simulink model "inverter_synth"  (R2020a)
settings: Solver=VariableStepAuto  StartTime=0.0  StopTime=0.75  MaxStep=0.001  RelTol=1e-4  EnableMultiTasking=on
model workspace (MAT data in the model file):
  f0 = 50
undefined symbols (not defined in the file): L, Lf, R, ron
libraries: powerlib x34, simulink_extras x9, powerlib_meascontrol x6, eeTransforms x5, simulink x5
settings Model: Creator=vm-user  LastModifiedBy=suku
settings DataIOCC: LimitDataPoints=on  SaveOutput=off  SaveTime=off  ReturnWorkspaceOutputs=off
settings OptimizationCC: ExpressionDepthLimit=2147483647  LifeSpan=1
settings DebuggingCC: UnderspecifiedInitializationDetection=Classic  MergeDetectMultiDrivingBlocksExec=none  FcnCallInpInsideContextMsg=warning  AllowSymbolicDim=off  StateNameClashWarn=warning  SFUnexpectedBacktrackingDiag=warning  SFNoUnconditionalDefaultTransitionDiag=warning  SFExecutionAtInitializationDiag=none  ArithmeticOperatorsInVariantConditions=warning
settings SFSimCC: SimUseLocalCustomCode=off  CustomCodeUndefinedFunction=UseInterfaceOnly
settings RTWCC: RTWUseLocalCustomCode=off
settings CodeAppCC: StateflowObjectComments=on
settings GRTTargetCC: TargetLangStandard=C89/C90 (ANSI)  CombineOutputUpdateFcns=off  GRTInterface=on

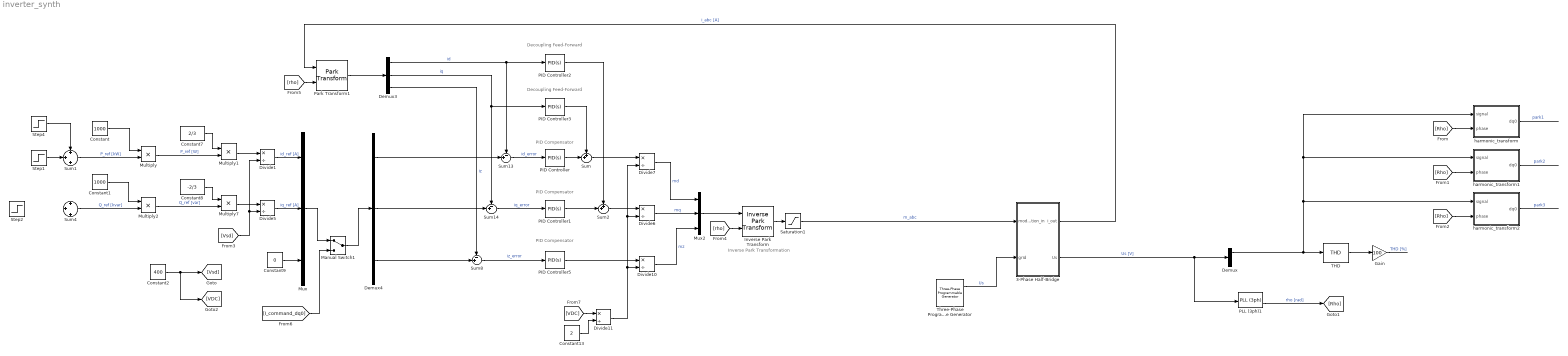
== system inverter_synth ==
  note: PID Compensator
  note: Decoupling Feed-Forward
  note: PID Compensator
  note: Decoupling Feed-Forward
  note: Inverse Park Transformation
  note: PID Compensator
  3-Phase Half-Bridge : Subsystem
  Constant : Constant  Value=1000
  Constant1 : Constant  Value=1000
  Constant13 : Constant  Value=2
  Constant2 : Constant  Value=400
  Constant7 : Constant  Value=2/3
  Constant8 : Constant  Value=-2/3
  Constant9 : Constant  Value=0
  Demux : Demux  Outputs=3
  Demux3 : Demux  Outputs=3
  Demux4 : Demux  Outputs=3
  Divide{1,5..7,10..11} (6 alike) : Product  Inputs=*/
  Gain : Gain  Gain=100
  Inverse Park Transform : eeTransforms/Inverse Park Transform  AxisAlignment=Q-axis  PowerInvariant=off
  Manual Switch1 : ManualSwitch
  Multiply{,1..2,7} (4 alike) : Product
  Mux : Mux  Inputs=3
  Mux2 : Mux  Inputs=3
  PID Controller : simulink/Continuous/PID Controller  Controller=PID  Form=Parallel  TimeDomain=Continuous-time  UseExternalTs=off  SampleTime=-1  IntegratorMethod=Forward Euler  FilterMethod=Forward Euler  ControllerParametersSource=internal  P=1  I=100  D=0.25  UseFilter=on  N=100  TunerSelectOption=Transfer Function Based (PID Tuner App)  InitialConditionSource=internal  InitialConditionForIntegrator=0  InitialConditionForFilter=0  DifferentiatorICPrevScaledInput=0  ExternalReset=none  TrackingMode=off  Kt=1  LimitOutput=off  UpperSaturationLimit=inf  LowerSaturationLimit=-inf  LinearizeAsGain=on  AntiWindupMode=none  Kb=1  POutMin=[]  POutMax=[]  IOutMin=[]  IOutMax=[]  DOutMin=[]  DOutMax=[]  NOutMin=[]  NOutMax=[]  SumOutMin=[]  SumOutMax=[]  SaturationOutMin=[]  SaturationOutMax=[]  PParamMin=[]  PParamMax=[]  IParamMin=[]  IParamMax=[]  DParamMin=[]  DParamMax=[]  NParamMin=[]  NParamMax=[]  KbParamMin=[]  KbParamMax=[]  KtParamMin=[]  KtParamMax=[]  KbOutMin=[]  KbOutMax=[]  KtOutMin=[]  KtOutMax=[]  IntegratorOutMin=[]  IntegratorOutMax=[]  FilterOutMin=[]  FilterOutMax=[]  SumI1OutMin=[]  SumI1OutMax=[]  SumI2OutMin=[]  SumI2OutMax=[]  SumI3OutMin=[]  SumI3OutMax=[]  SumI4OutMin=[]  SumI4OutMax=[]  SumDOutMin=[]  SumDOutMax=[]  DifferentiatorOutMin=[]  DifferentiatorOutMax=[]  FilterDiffOutCoefMin=[]  FilterDiffOutCoefMax=[]  ReciprocalOutMin=[]  ReciprocalOutMax=[]  SumDenOutMin=[]  SumDenOutMax=[]  SumNumOutMin=[]  SumNumOutMax=[]  DivideOutMin=[]  DivideOutMax=[]  UdiffTsProdOutMin=[]  UdiffTsProdOutMax=[]  NTsProdOutMin=[]  NTsProdOutMax=[]  UintegralTsProdOutMin=[]  UintegralTsProdOutMax=[]  UngainTsProdOutMin=[]  UngainTsProdOutMax=[]  IntegratorContinuousStateAttributes=''  IntegratorStateMustResolveToSignalObject=off  IntegratorRTWStateStorageClass=Auto  FilterContinuousStateAttributes=''  FilterStateMustResolveToSignalObject=off  FilterRTWStateStorageClass=Auto  ParallelPVariant=InternalParameters  IdealPVariant=Disabled  IVariant=InternalParameters  DVariant=InternalParameters  IntegratorVariant=Continuous  SatVariant=Disabled  AWVariant=Passthrough  PCopyVariant=Disabled  TRVariant=Disabled  FdbkBlocksVariant=Forward  IdealPFdbkVariant=Disabled  SatFdbkVariant=Disabled  DerivativeFilterVariant=ContFilter  NVariant=InternalParameters  NCopyVariant=Disabled  FilterICVariant=InternalICsFilter  IntegratorICVariant=InternalICs  ExternalResetVariant=Disabled  TRSumVariant=Passthrough  SumFdbkVariant=Disabled  SumVariant=Sum_PID  TsampFilterVariant=InternalTs  TsampNgainVariant=Passthrough  TsampIntegralVariant=Passthrough
  PID Controller1 : simulink/Continuous/PID Controller  Controller=PID  Form=Parallel  TimeDomain=Continuous-time  UseExternalTs=off  SampleTime=-1  IntegratorMethod=Forward Euler  FilterMethod=Forward Euler  ControllerParametersSource=internal  P=1  I=100  D=0.25  UseFilter=on  N=100  TunerSelectOption=Transfer Function Based (PID Tuner App)  InitialConditionSource=internal  InitialConditionForIntegrator=0  InitialConditionForFilter=0  DifferentiatorICPrevScaledInput=0  ExternalReset=none  TrackingMode=off  Kt=1  LimitOutput=off  UpperSaturationLimit=inf  LowerSaturationLimit=-inf  LinearizeAsGain=on  AntiWindupMode=none  Kb=1  POutMin=[]  POutMax=[]  IOutMin=[]  IOutMax=[]  DOutMin=[]  DOutMax=[]  NOutMin=[]  NOutMax=[]  SumOutMin=[]  SumOutMax=[]  SaturationOutMin=[]  SaturationOutMax=[]  PParamMin=[]  PParamMax=[]  IParamMin=[]  IParamMax=[]  DParamMin=[]  DParamMax=[]  NParamMin=[]  NParamMax=[]  KbParamMin=[]  KbParamMax=[]  KtParamMin=[]  KtParamMax=[]  KbOutMin=[]  KbOutMax=[]  KtOutMin=[]  KtOutMax=[]  IntegratorOutMin=[]  IntegratorOutMax=[]  FilterOutMin=[]  FilterOutMax=[]  SumI1OutMin=[]  SumI1OutMax=[]  SumI2OutMin=[]  SumI2OutMax=[]  SumI3OutMin=[]  SumI3OutMax=[]  SumI4OutMin=[]  SumI4OutMax=[]  SumDOutMin=[]  SumDOutMax=[]  DifferentiatorOutMin=[]  DifferentiatorOutMax=[]  FilterDiffOutCoefMin=[]  FilterDiffOutCoefMax=[]  ReciprocalOutMin=[]  ReciprocalOutMax=[]  SumDenOutMin=[]  SumDenOutMax=[]  SumNumOutMin=[]  SumNumOutMax=[]  DivideOutMin=[]  DivideOutMax=[]  UdiffTsProdOutMin=[]  UdiffTsProdOutMax=[]  NTsProdOutMin=[]  NTsProdOutMax=[]  UintegralTsProdOutMin=[]  UintegralTsProdOutMax=[]  UngainTsProdOutMin=[]  UngainTsProdOutMax=[]  IntegratorContinuousStateAttributes=''  IntegratorStateMustResolveToSignalObject=off  IntegratorRTWStateStorageClass=Auto  FilterContinuousStateAttributes=''  FilterStateMustResolveToSignalObject=off  FilterRTWStateStorageClass=Auto  ParallelPVariant=InternalParameters  IdealPVariant=Disabled  IVariant=InternalParameters  DVariant=InternalParameters  IntegratorVariant=Continuous  SatVariant=Disabled  AWVariant=Passthrough  PCopyVariant=Disabled  TRVariant=Disabled  FdbkBlocksVariant=Forward  IdealPFdbkVariant=Disabled  SatFdbkVariant=Disabled  DerivativeFilterVariant=ContFilter  NVariant=InternalParameters  NCopyVariant=Disabled  FilterICVariant=InternalICsFilter  IntegratorICVariant=InternalICs  ExternalResetVariant=Disabled  TRSumVariant=Passthrough  SumFdbkVariant=Disabled  SumVariant=Sum_PID  TsampFilterVariant=InternalTs  TsampNgainVariant=Passthrough  TsampIntegralVariant=Passthrough
  PID Controller2 : simulink/Continuous/PID Controller  Controller=PID  Form=Parallel  TimeDomain=Continuous-time  UseExternalTs=off  SampleTime=-1  IntegratorMethod=Forward Euler  FilterMethod=Forward Euler  ControllerParametersSource=internal  P=0.22  I=0  D=0  UseFilter=on  N=100  TunerSelectOption=Transfer Function Based (PID Tuner App)  InitialConditionSource=internal  InitialConditionForIntegrator=0  InitialConditionForFilter=0  DifferentiatorICPrevScaledInput=0  ExternalReset=none  TrackingMode=off  Kt=1  LimitOutput=off  UpperSaturationLimit=inf  LowerSaturationLimit=-inf  LinearizeAsGain=on  AntiWindupMode=none  Kb=1  POutMin=[]  POutMax=[]  IOutMin=[]  IOutMax=[]  DOutMin=[]  DOutMax=[]  NOutMin=[]  NOutMax=[]  SumOutMin=[]  SumOutMax=[]  SaturationOutMin=[]  SaturationOutMax=[]  PParamMin=[]  PParamMax=[]  IParamMin=[]  IParamMax=[]  DParamMin=[]  DParamMax=[]  NParamMin=[]  NParamMax=[]  KbParamMin=[]  KbParamMax=[]  KtParamMin=[]  KtParamMax=[]  KbOutMin=[]  KbOutMax=[]  KtOutMin=[]  KtOutMax=[]  IntegratorOutMin=[]  IntegratorOutMax=[]  FilterOutMin=[]  FilterOutMax=[]  SumI1OutMin=[]  SumI1OutMax=[]  SumI2OutMin=[]  SumI2OutMax=[]  SumI3OutMin=[]  SumI3OutMax=[]  SumI4OutMin=[]  SumI4OutMax=[]  SumDOutMin=[]  SumDOutMax=[]  DifferentiatorOutMin=[]  DifferentiatorOutMax=[]  FilterDiffOutCoefMin=[]  FilterDiffOutCoefMax=[]  ReciprocalOutMin=[]  ReciprocalOutMax=[]  SumDenOutMin=[]  SumDenOutMax=[]  SumNumOutMin=[]  SumNumOutMax=[]  DivideOutMin=[]  DivideOutMax=[]  UdiffTsProdOutMin=[]  UdiffTsProdOutMax=[]  NTsProdOutMin=[]  NTsProdOutMax=[]  UintegralTsProdOutMin=[]  UintegralTsProdOutMax=[]  UngainTsProdOutMin=[]  UngainTsProdOutMax=[]  IntegratorContinuousStateAttributes=''  IntegratorStateMustResolveToSignalObject=off  IntegratorRTWStateStorageClass=Auto  FilterContinuousStateAttributes=''  FilterStateMustResolveToSignalObject=off  FilterRTWStateStorageClass=Auto  ParallelPVariant=InternalParameters  IdealPVariant=Disabled  IVariant=InternalParameters  DVariant=InternalParameters  IntegratorVariant=Continuous  SatVariant=Disabled  AWVariant=Passthrough  PCopyVariant=Disabled  TRVariant=Disabled  FdbkBlocksVariant=Forward  IdealPFdbkVariant=Disabled  SatFdbkVariant=Disabled  DerivativeFilterVariant=ContFilter  NVariant=InternalParameters  NCopyVariant=Disabled  FilterICVariant=InternalICsFilter  IntegratorICVariant=InternalICs  ExternalResetVariant=Disabled  TRSumVariant=Passthrough  SumFdbkVariant=Disabled  SumVariant=Sum_PID  TsampFilterVariant=InternalTs  TsampNgainVariant=Passthrough  TsampIntegralVariant=Passthrough
  PID Controller3 : simulink/Continuous/PID Controller  Controller=PID  Form=Parallel  TimeDomain=Continuous-time  UseExternalTs=off  SampleTime=-1  IntegratorMethod=Forward Euler  FilterMethod=Forward Euler  ControllerParametersSource=internal  P=-0.22  I=0  D=0  UseFilter=on  N=100  TunerSelectOption=Transfer Function Based (PID Tuner App)  InitialConditionSource=internal  InitialConditionForIntegrator=0  InitialConditionForFilter=0  DifferentiatorICPrevScaledInput=0  ExternalReset=none  TrackingMode=off  Kt=1  LimitOutput=off  UpperSaturationLimit=inf  LowerSaturationLimit=-inf  LinearizeAsGain=on  AntiWindupMode=none  Kb=1  POutMin=[]  POutMax=[]  IOutMin=[]  IOutMax=[]  DOutMin=[]  DOutMax=[]  NOutMin=[]  NOutMax=[]  SumOutMin=[]  SumOutMax=[]  SaturationOutMin=[]  SaturationOutMax=[]  PParamMin=[]  PParamMax=[]  IParamMin=[]  IParamMax=[]  DParamMin=[]  DParamMax=[]  NParamMin=[]  NParamMax=[]  KbParamMin=[]  KbParamMax=[]  KtParamMin=[]  KtParamMax=[]  KbOutMin=[]  KbOutMax=[]  KtOutMin=[]  KtOutMax=[]  IntegratorOutMin=[]  IntegratorOutMax=[]  FilterOutMin=[]  FilterOutMax=[]  SumI1OutMin=[]  SumI1OutMax=[]  SumI2OutMin=[]  SumI2OutMax=[]  SumI3OutMin=[]  SumI3OutMax=[]  SumI4OutMin=[]  SumI4OutMax=[]  SumDOutMin=[]  SumDOutMax=[]  DifferentiatorOutMin=[]  DifferentiatorOutMax=[]  FilterDiffOutCoefMin=[]  FilterDiffOutCoefMax=[]  ReciprocalOutMin=[]  ReciprocalOutMax=[]  SumDenOutMin=[]  SumDenOutMax=[]  SumNumOutMin=[]  SumNumOutMax=[]  DivideOutMin=[]  DivideOutMax=[]  UdiffTsProdOutMin=[]  UdiffTsProdOutMax=[]  NTsProdOutMin=[]  NTsProdOutMax=[]  UintegralTsProdOutMin=[]  UintegralTsProdOutMax=[]  UngainTsProdOutMin=[]  UngainTsProdOutMax=[]  IntegratorContinuousStateAttributes=''  IntegratorStateMustResolveToSignalObject=off  IntegratorRTWStateStorageClass=Auto  FilterContinuousStateAttributes=''  FilterStateMustResolveToSignalObject=off  FilterRTWStateStorageClass=Auto  ParallelPVariant=InternalParameters  IdealPVariant=Disabled  IVariant=InternalParameters  DVariant=InternalParameters  IntegratorVariant=Continuous  SatVariant=Disabled  AWVariant=Passthrough  PCopyVariant=Disabled  TRVariant=Disabled  FdbkBlocksVariant=Forward  IdealPFdbkVariant=Disabled  SatFdbkVariant=Disabled  DerivativeFilterVariant=ContFilter  NVariant=InternalParameters  NCopyVariant=Disabled  FilterICVariant=InternalICsFilter  IntegratorICVariant=InternalICs  ExternalResetVariant=Disabled  TRSumVariant=Passthrough  SumFdbkVariant=Disabled  SumVariant=Sum_PID  TsampFilterVariant=InternalTs  TsampNgainVariant=Passthrough  TsampIntegralVariant=Passthrough
  PID Controller5 : simulink/Continuous/PID Controller  Controller=PID  Form=Parallel  TimeDomain=Continuous-time  UseExternalTs=off  SampleTime=-1  IntegratorMethod=Forward Euler  FilterMethod=Forward Euler  ControllerParametersSource=internal  P=1  I=100  D=0.25  UseFilter=on  N=100  TunerSelectOption=Transfer Function Based (PID Tuner App)  InitialConditionSource=internal  InitialConditionForIntegrator=0  InitialConditionForFilter=0  DifferentiatorICPrevScaledInput=0  ExternalReset=none  TrackingMode=off  Kt=1  LimitOutput=off  UpperSaturationLimit=inf  LowerSaturationLimit=-inf  LinearizeAsGain=on  AntiWindupMode=none  Kb=1  POutMin=[]  POutMax=[]  IOutMin=[]  IOutMax=[]  DOutMin=[]  DOutMax=[]  NOutMin=[]  NOutMax=[]  SumOutMin=[]  SumOutMax=[]  SaturationOutMin=[]  SaturationOutMax=[]  PParamMin=[]  PParamMax=[]  IParamMin=[]  IParamMax=[]  DParamMin=[]  DParamMax=[]  NParamMin=[]  NParamMax=[]  KbParamMin=[]  KbParamMax=[]  KtParamMin=[]  KtParamMax=[]  KbOutMin=[]  KbOutMax=[]  KtOutMin=[]  KtOutMax=[]  IntegratorOutMin=[]  IntegratorOutMax=[]  FilterOutMin=[]  FilterOutMax=[]  SumI1OutMin=[]  SumI1OutMax=[]  SumI2OutMin=[]  SumI2OutMax=[]  SumI3OutMin=[]  SumI3OutMax=[]  SumI4OutMin=[]  SumI4OutMax=[]  SumDOutMin=[]  SumDOutMax=[]  DifferentiatorOutMin=[]  DifferentiatorOutMax=[]  FilterDiffOutCoefMin=[]  FilterDiffOutCoefMax=[]  ReciprocalOutMin=[]  ReciprocalOutMax=[]  SumDenOutMin=[]  SumDenOutMax=[]  SumNumOutMin=[]  SumNumOutMax=[]  DivideOutMin=[]  DivideOutMax=[]  UdiffTsProdOutMin=[]  UdiffTsProdOutMax=[]  NTsProdOutMin=[]  NTsProdOutMax=[]  UintegralTsProdOutMin=[]  UintegralTsProdOutMax=[]  UngainTsProdOutMin=[]  UngainTsProdOutMax=[]  IntegratorContinuousStateAttributes=''  IntegratorStateMustResolveToSignalObject=off  IntegratorRTWStateStorageClass=Auto  FilterContinuousStateAttributes=''  FilterStateMustResolveToSignalObject=off  FilterRTWStateStorageClass=Auto  ParallelPVariant=InternalParameters  IdealPVariant=Disabled  IVariant=InternalParameters  DVariant=InternalParameters  IntegratorVariant=Continuous  SatVariant=Disabled  AWVariant=Passthrough  PCopyVariant=Disabled  TRVariant=Disabled  FdbkBlocksVariant=Forward  IdealPFdbkVariant=Disabled  SatFdbkVariant=Disabled  DerivativeFilterVariant=ContFilter  NVariant=InternalParameters  NCopyVariant=Disabled  FilterICVariant=InternalICsFilter  IntegratorICVariant=InternalICs  ExternalResetVariant=Disabled  TRSumVariant=Passthrough  SumFdbkVariant=Disabled  SumVariant=Sum_PID  TsampFilterVariant=InternalTs  TsampNgainVariant=Passthrough  TsampIntegralVariant=Passthrough
  PLL (3ph)1 : powerlib_meascontrol/PLL/PLL (3ph)  Fmin=40  Par_Init=[0, 50]  ParK=[180, 3200, 1]  TcD=1e-4  MaxRateChangeFreq=12  FilterCutOffFreq=25  Ts=0  AGC=on
  Park Transform1 : eeTransforms/Park Transform  AxisAlignment=Q-axis  PowerInvariant=off
  Saturation1 : Saturate  UpperLimit=1  LowerLimit=-1
  Step1 : Step  Time=0.1  After=8  SampleTime=0
  Step2 : Step  Time=0.5  After=6  SampleTime=0
  Step4 : Step  Time=0.5  After=-4  SampleTime=0
  Sum : Sum  Inputs=++|
  Sum1 : Sum  Inputs=+|+|+
  Sum13 : Sum  Inputs=-+|
  Sum14 : Sum  Inputs=-+|
  Sum2 : Sum  Inputs=++|
  Sum4 : Sum  Inputs=+|+|+
  Sum8 : Sum  Inputs=-+|
  THD : powerlib_meascontrol/Measurements/THD  Freq=50  Ts=0
  Three-Phase Programmable Generator : powerlib_meascontrol/Pulse & Signal Generators/Three-Phase Programmable Generator  Par_Vps=[231, 0, 50]  VariationEntity=None  VariationType=Ramp  VariationStep=-0.5  VariationRate=10  VariationMag=0.3  VariationFreq=2  Par_Timing_Variation="[0.2  1.2]"  SinglePhase=on  Yampli=[1 0.2 1.2 1.0]  Xtime=[0 0.1 0.15 0.2]  HarmonicGeneration=on  Par_HarmoA="[3  50  25 0]"  Par_HarmoB="[5  30  -42  2]"  Par_Timing_Harmo="[ 0.05  99]"  Ts=0
      settings: SourceProductBaseCode=PS
  harmonic_transform : Subsystem  mask{f0=50, h=1}
      mask prompts: f0 "fundamental frequency"; h "harmonic number"
  harmonic_transform1 : Subsystem  mask{f0=50, h=3}
      mask prompts: f0 "fundamental frequency"; h "harmonic number"
  harmonic_transform2 : Subsystem  mask{f0=50, h=5}
      mask prompts: f0 "fundamental frequency"; h "harmonic number"
  wires:
  PLL (3ph)1/2 -> [Rho]  "rho [rad]"
  harmonic_transform/1(dq0) -> ?  "park1"
  [Rho] -> harmonic_transform/2(phase)
  [Rho] -> harmonic_transform1/2(phase)
  harmonic_transform1/1(dq0) -> ?  "park2"
  harmonic_transform2/1(dq0) -> ?  "park3"
  [Rho] -> harmonic_transform2/2(phase)
  Demux/1 -> harmonic_transform1/1(signal), harmonic_transform/1(signal), harmonic_transform2/1(signal), THD/1
  THD/1 -> Gain/1
  Gain/1 -> ?  "THD [%]"
  3-Phase Half-Bridge/2(Us) -> PLL (3ph)1/1, Demux/1  "Us [V]"
  Sum4/1 -> Multiply2/2  "Q_ref [kvar]"
  Demux4/1 -> Sum13/2
  Divide7/1 -> Mux2/1  "md"
  PID Controller2/1 -> Sum2/1
  Demux4/2 -> Sum14/2
  Demux3/3 -> Sum8/1  "iz"
  Sum8/1 -> PID Controller5/1  "iz_error"
  Constant7/1 -> Multiply1/1
  Constant9/1 -> Mux/3
  Sum14/1 -> PID Controller1/1  "iq_error"
  Divide1/1 -> Mux/1  "id_ref [A]"
  Sum2/1 -> Divide6/1
  Divide10/1 -> Mux2/3  "mz"
  Multiply7/1 -> Divide5/1
  [rho] -> Park Transform1/2
  Sum/1 -> Divide7/1
  PID Controller5/1 -> Divide10/1
  Manual Switch1/1 -> Demux4/1
  Divide6/1 -> Mux2/2  "mq"
  [rho] -> Inverse Park Transform/2
  Step1/1 -> Sum1/2
  PID Controller1/1 -> Sum2/2
  PID Controller3/1 -> Sum/1
  Step4/1 -> Sum1/1
  [VDC] -> Divide11/1
  3-Phase Half-Bridge/1(i_out) -> Park Transform1/1  "i_abc [A]"
  Demux3/2 -> Sum14/1, PID Controller3/1  "iq"
  Inverse Park Transform/1 -> Saturation1/1
  Divide11/1 -> Divide10/2, Divide7/2, Divide6/2
  Constant13/1 -> Divide11/2
  Constant1/1 -> Multiply2/1
  Multiply2/1 -> Multiply7/2  "Q_ref [var]"
  [Vsd] -> Divide1/2, Divide5/2
  Saturation1/1 -> 3-Phase Half-Bridge/1(modulation_in)  "m_abc"
  Multiply/1 -> Multiply1/2  "P_ref [W]"
  Demux3/1 -> Sum13/1, PID Controller2/1  "id"
  Mux/1 -> Manual Switch1/1
  Multiply1/1 -> Divide1/1
  Demux4/3 -> Sum8/2
  Constant/1 -> Multiply/1
  Sum13/1 -> PID Controller/1  "id_error"
  Divide5/1 -> Mux/2  "iq_ref [A]"
  Mux2/1 -> Inverse Park Transform/1
  [I_command_dq0] -> Manual Switch1/2
  Sum1/1 -> Multiply/2  "P_ref [kW]"
  Constant8/1 -> Multiply7/1
  PID Controller/1 -> Sum/2
  Park Transform1/1 -> Demux3/1
  Three-Phase Programmable Generator/1 -> 3-Phase Half-Bridge/2(grid)  "Us"
  Constant2/1 -> [VDC], [Vsd]

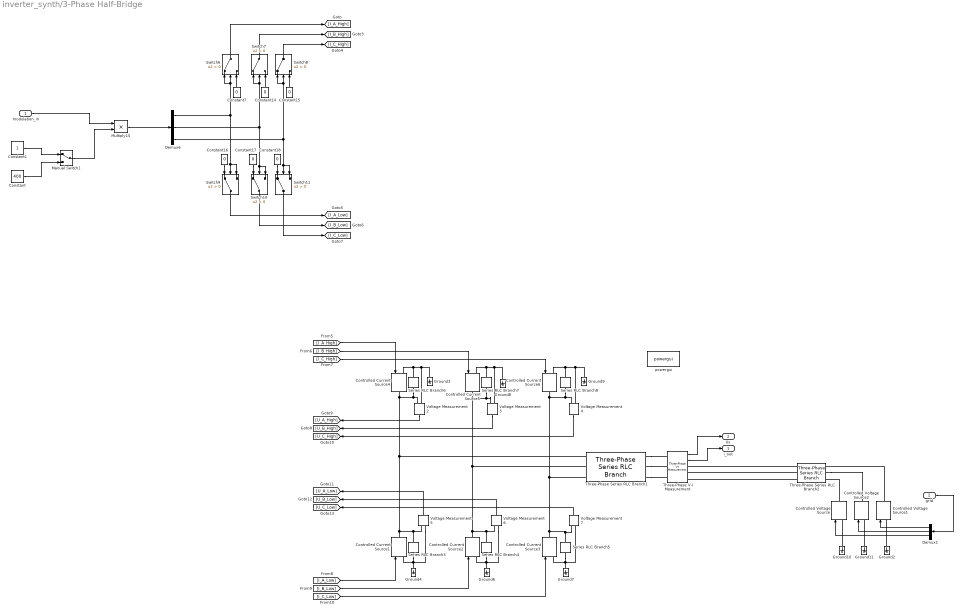
== system inverter_synth/3-Phase Half-Bridge ==
  modulation_in : Inport
  grid : Inport  Port=2
  Constant : Constant  Value=400
  Constant1 : Constant
  Constant{7,14..18} (6 alike) : Constant  Value=0
  Controlled Current Source{1..6} (6 alike) : powerlib/Electrical Sources/Controlled Current Source  Initialize=on  Source_Type=DC  Amplitude=0  Phase=0  Frequency=0  Measurements=None
  Controlled Voltage Source : powerlib/Electrical Sources/Controlled Voltage Source  Initialize=on  Source_Type=DC  Amplitude=0  Phase=0  Frequency=0  Measurements=None
  Controlled Voltage Source1 : powerlib/Electrical Sources/Controlled Voltage Source  Initialize=on  Source_Type=DC  Amplitude=0  Phase=0  Frequency=0  Measurements=None
  Controlled Voltage Source2 : powerlib/Electrical Sources/Controlled Voltage Source  Initialize=on  Source_Type=DC  Amplitude=0  Phase=0  Frequency=0  Measurements=None
  Demux1 : Demux  Outputs=3
  Demux6 : Demux  Outputs=3
  Ground{2..4,6..11} (9 alike) : powerlib/Elements/Ground  LConnTagsString=a
  Manual Switch1 : ManualSwitch
  Multiply15 : Product
  Series RLC Branch{3..8} (6 alike) : powerlib/Elements/Series RLC Branch  LConnTagsString=__new0  RConnTagsString=__new0  BranchType=R  Resistance=5000  Inductance=1e-3  SetiL0=off  InitialCurrent=0  Capacitance=47000e-6  Setx0=on  InitialVoltage=300  Measurements=None
  Switch{6..11} (6 alike) : Switch  Criteria=u2 > Threshold
  Three-Phase Series RLC Branch1 : powerlib/Elements/Three-Phase Series RLC Branch  LConnTagsString=A|B|C  RConnTagsString=A|B|C  BranchType=RL  Resistance=R + ron  Inductance=L  Capacitance=1e-6  Measurements=None
  Three-Phase Series RLC Branch2 : powerlib/Elements/Three-Phase Series RLC Branch  LConnTagsString=A|B|C  RConnTagsString=A|B|C  BranchType=RL  Resistance=1  Inductance=Lf  Capacitance=1e-6  Measurements=None
  Three-Phase V-I Measurement : powerlib/Measurements/Three-Phase V-I Measurement  VoltageMeasurement=phase-to-ground  SetLabelV=off  LabelV=Vabc  Vpu=off  VpuLL=off  CurrentMeasurement=yes  SetLabelI=off  LabelI=Iabc  Ipu=off  Pbase=100e6  Vbase=500e3  OutputType=Complex  PhasorSimulation=off  PSBequivalent=0
  Voltage Measurement{2..7} (6 alike) : powerlib/Measurements/Voltage Measurement  PhasorSimulation=off  OutputType=Magnitude  PSBequivalent=0
  powergui : powerlib/powergui  Priority=1  SimulationMode=Continuous  SampleTime=50e-6  frequency=60  Iterations=50  frequencyindice=0  Pbase=100e6  ErrMax=1e-4  UnitsV=kV  UnitsW=MW  buscounter=0  FunctionMessages=off  echomessages=off  EnableUseOfTLC=off  CurrentSourceSwitches=off  DisableSnubberDevices=off  DisableRonSwitches=off  DisableVfSwitches=off  DisplayEquations=off  AutomaticDiscreteSolvers=off  SolverType=Tustin/Backward Euler (TBE)  Interpol=off  ExternalGateDelay=off  methode=off  Ts=100  x0status=blocks  SPID=on  SwTol=0  HookPort=off  NonlinearTolerance=1e-4  nMaxIteration=100  ContinueOnMaxIteration=off  RestoreLinks=warning  ResistiveCurrentMeasurement=off  Frange=[0:2:500]  Ylog=off  Xlog=on  ShowGrid=off  save=off  variable=ZData  structure=0  ZoomFFT=off  StartTime=0.0  cycles=1  DisplayStyle=1  fundamental=60  FreqAxis=off  MaxFrequency=1000  frequencyindicesteady=1  RmsSteady=1  display=off
  i_out : Outport  VectorParamsAs1DForOutWhenUnconnected=off
  Us : Outport  Port=2  VectorParamsAs1DForOutWhenUnconnected=off
  wires:
  Constant18/1 -> Switch11/1
  Constant7/1 -> Switch6/3
  Constant16/1 -> Switch9/1
  Constant14/1 -> Switch7/3
  Constant17/1 -> Switch10/1
  Three-Phase V-I Measurement/2 -> i_out/1
  Constant15/1 -> Switch8/3
  Three-Phase V-I Measurement/1 -> Us/1
  modulation_in/1 -> Multiply15/1
  [I_A_High] -> Controlled Current Source4/1
  [I_B_High] -> Controlled Current Source5/1
  [I_C_High] -> Controlled Current Source6/1
  [I_B_Low] -> Controlled Current Source2/1
  [I_C_Low] -> Controlled Current Source3/1
  [I_A_Low] -> Controlled Current Source1/1
  Voltage Measurement2/1 -> [U_A_High]
  Voltage Measurement3/1 -> [U_B_High]
  Voltage Measurement4/1 -> [U_C_High]
  Voltage Measurement5/1 -> [U_A_Low]
  Voltage Measurement6/1 -> [U_B_Low]
  Voltage Measurement7/1 -> [U_C_Low]
  Switch8/1 -> [I_C_High]
  Switch7/1 -> [I_B_High]
  Switch6/1 -> [I_A_High]
  Switch11/1 -> [I_C_Low]
  Switch10/1 -> [I_B_Low]
  Switch9/1 -> [I_A_Low]
  Demux6/1 -> Switch6/1, Switch6/2, Switch9/3, Switch9/2
  Demux6/2 -> Switch7/1, Switch7/2, Switch10/3, Switch10/2
  Demux6/3 -> Switch11/3, Switch11/2, Switch8/1, Switch8/2
  Manual Switch1/1 -> Multiply15/2
  Constant/1 -> Manual Switch1/2
  Demux1/3 -> Controlled Voltage Source/1
  Demux1/2 -> Controlled Voltage Source2/1
  Demux1/1 -> Controlled Voltage Source1/1
  grid/1 -> Demux1/1
  Multiply15/1 -> Demux6/1
  Constant1/1 -> Manual Switch1/1
  connections:
  Controlled Current Source1/RConn1 -- Voltage Measurement5/LConn2 -- Series RLC Branch3/LConn1 -- Three-Phase Series RLC Branch1/LConn1 -- Voltage Measurement2/LConn2 -- Series RLC Branch6/RConn1 -- Controlled Current Source4/RConn1
  Controlled Current Source2/RConn1 -- Voltage Measurement6/LConn2 -- Series RLC Branch4/LConn1 -- Three-Phase Series RLC Branch1/LConn2 -- Voltage Measurement3/LConn2 -- Series RLC Branch7/RConn1 -- Controlled Current Source5/RConn1
  Controlled Current Source3/RConn1 -- Voltage Measurement7/LConn2 -- Series RLC Branch5/LConn1 -- Voltage Measurement4/LConn2 -- Series RLC Branch8/RConn1 -- Controlled Current Source6/RConn1 -- Three-Phase Series RLC Branch1/LConn3
  Three-Phase Series RLC Branch2/LConn1 -- Three-Phase V-I Measurement/RConn1
  Three-Phase Series RLC Branch2/LConn2 -- Three-Phase V-I Measurement/RConn2
  Three-Phase Series RLC Branch2/LConn3 -- Three-Phase V-I Measurement/RConn3
  Series RLC Branch4/RConn1 -- Voltage Measurement6/LConn1 -- Ground6/LConn1 -- Controlled Current Source2/LConn1
  Series RLC Branch3/RConn1 -- Voltage Measurement5/LConn1 -- Ground4/LConn1 -- Controlled Current Source1/LConn1
  Controlled Current Source5/LConn1 -- Ground8/LConn1 -- Voltage Measurement3/LConn1 -- Series RLC Branch7/LConn1
  Series RLC Branch5/RConn1 -- Ground7/LConn1 -- Controlled Current Source3/LConn1 -- Voltage Measurement7/LConn1
  Ground3/LConn1 -- Controlled Current Source4/LConn1 -- Series RLC Branch6/LConn1 -- Voltage Measurement2/LConn1
  Voltage Measurement4/LConn1 -- Controlled Current Source6/LConn1 -- Series RLC Branch8/LConn1 -- Ground9/LConn1
  Three-Phase Series RLC Branch1/RConn1 -- Three-Phase V-I Measurement/LConn1
  Three-Phase Series RLC Branch1/RConn2 -- Three-Phase V-I Measurement/LConn2
  Three-Phase Series RLC Branch1/RConn3 -- Three-Phase V-I Measurement/LConn3
  Three-Phase Series RLC Branch2/RConn2 -- Controlled Voltage Source2/RConn1
  Controlled Voltage Source/RConn1 -- Three-Phase Series RLC Branch2/RConn3
  Ground11/LConn1 -- Controlled Voltage Source2/LConn1
  Ground2/LConn1 -- Controlled Voltage Source1/LConn1
  Ground10/LConn1 -- Controlled Voltage Source/LConn1
  Controlled Voltage Source1/RConn1 -- Three-Phase Series RLC Branch2/RConn1

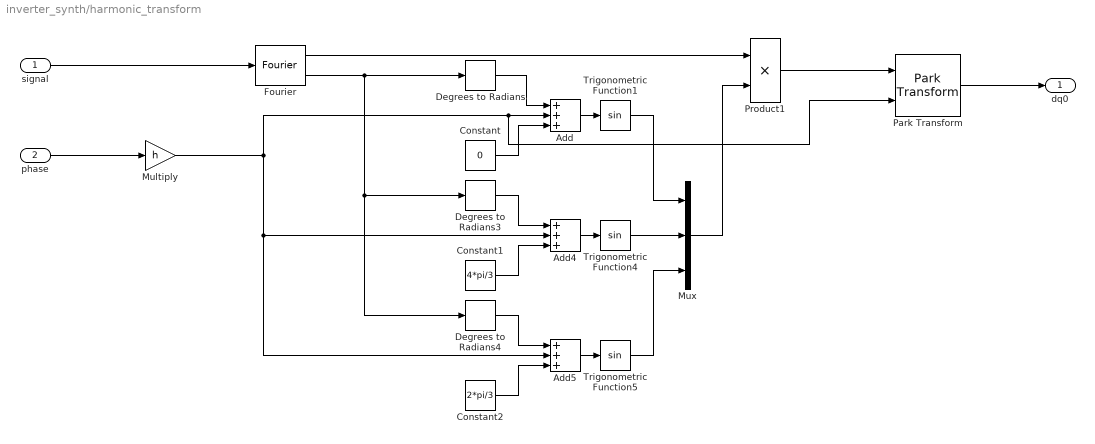
== system inverter_synth/harmonic_transform ==
  signal : Inport
  phase : Inport  Port=2
  Add : Sum  Inputs=+++
  Add4 : Sum  Inputs=+++
  Add5 : Sum  Inputs=+++
  Constant : Constant  Value=0
  Constant1 : Constant  Value=4*pi/3
  Constant2 : Constant  Value=2*pi/3
  Degrees to Radians : simulink_extras/Transformations/Degrees to Radians
  Degrees to Radians3 : simulink_extras/Transformations/Degrees to Radians
  Degrees to Radians4 : simulink_extras/Transformations/Degrees to Radians
  Fourier : powerlib_meascontrol/Measurements/Fourier  Freq=f0  n=h  InInit=[0, 0]  Ts=0
  Multiply : Gain  Gain=h
  Mux : Mux  Inputs=3
  Park Transform : eeTransforms/Park Transform  AxisAlignment=Q-axis  PowerInvariant=off
  Product1 : Product  RndMeth=Zero
  Trigonometric Function1 : Trigonometry
  Trigonometric Function4 : Trigonometry
  Trigonometric Function5 : Trigonometry
  dq0 : Outport
  wires:
  Add/1 -> Trigonometric Function1/1
  Multiply/1 -> Add5/2, Add4/2, Park Transform/2, Add/2
  Constant2/1 -> Add5/3
  Mux/1 -> Product1/2
  Fourier/1 -> Product1/1
  Degrees to Radians/1 -> Add/1
  Fourier/2 -> Degrees to Radians/1, Degrees to Radians3/1, Degrees to Radians4/1
  Degrees to Radians4/1 -> Add5/1
  Constant/1 -> Add/3
  Add5/1 -> Trigonometric Function5/1
  Product1/1 -> Park Transform/1
  Trigonometric Function5/1 -> Mux/3
  Trigonometric Function1/1 -> Mux/1
  Park Transform/1 -> dq0/1
  Add4/1 -> Trigonometric Function4/1
  Degrees to Radians3/1 -> Add4/1
  Constant1/1 -> Add4/3
  Trigonometric Function4/1 -> Mux/2
  signal/1 -> Fourier/1
  phase/1 -> Multiply/1

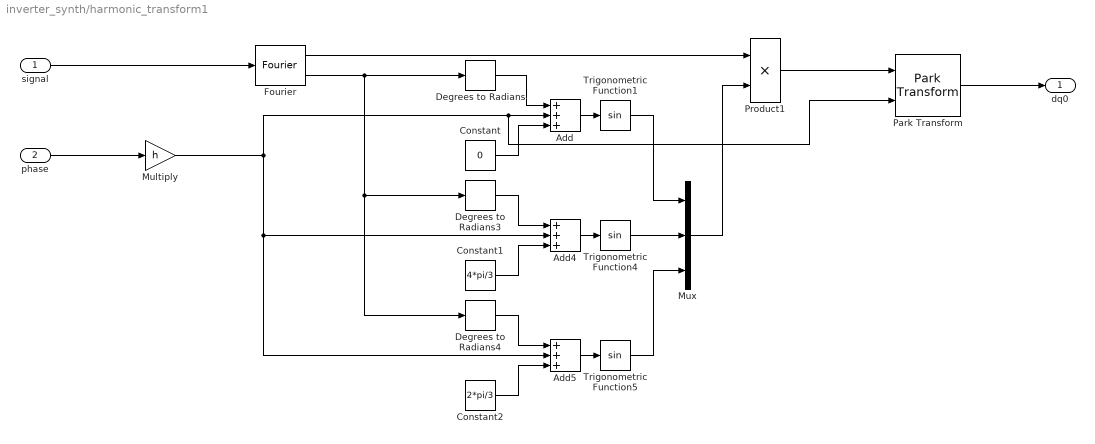
== system inverter_synth/harmonic_transform1 ==
  signal : Inport
  phase : Inport  Port=2
  Add : Sum  Inputs=+++
  Add4 : Sum  Inputs=+++
  Add5 : Sum  Inputs=+++
  Constant : Constant  Value=0
  Constant1 : Constant  Value=4*pi/3
  Constant2 : Constant  Value=2*pi/3
  Degrees to Radians : simulink_extras/Transformations/Degrees to Radians
  Degrees to Radians3 : simulink_extras/Transformations/Degrees to Radians
  Degrees to Radians4 : simulink_extras/Transformations/Degrees to Radians
  Fourier : powerlib_meascontrol/Measurements/Fourier  Freq=f0  n=h  InInit=[0, 0]  Ts=0
  Multiply : Gain  Gain=h
  Mux : Mux  Inputs=3
  Park Transform : eeTransforms/Park Transform  AxisAlignment=Q-axis  PowerInvariant=off
  Product1 : Product  RndMeth=Zero
  Trigonometric Function1 : Trigonometry
  Trigonometric Function4 : Trigonometry
  Trigonometric Function5 : Trigonometry
  dq0 : Outport
  wires:
  Add/1 -> Trigonometric Function1/1
  Multiply/1 -> Add5/2, Add4/2, Park Transform/2, Add/2
  Constant2/1 -> Add5/3
  Mux/1 -> Product1/2
  Fourier/1 -> Product1/1
  Degrees to Radians/1 -> Add/1
  Fourier/2 -> Degrees to Radians/1, Degrees to Radians3/1, Degrees to Radians4/1
  Degrees to Radians4/1 -> Add5/1
  Constant/1 -> Add/3
  Add5/1 -> Trigonometric Function5/1
  Product1/1 -> Park Transform/1
  Trigonometric Function5/1 -> Mux/3
  Trigonometric Function1/1 -> Mux/1
  Park Transform/1 -> dq0/1
  Add4/1 -> Trigonometric Function4/1
  Degrees to Radians3/1 -> Add4/1
  Constant1/1 -> Add4/3
  Trigonometric Function4/1 -> Mux/2
  signal/1 -> Fourier/1
  phase/1 -> Multiply/1

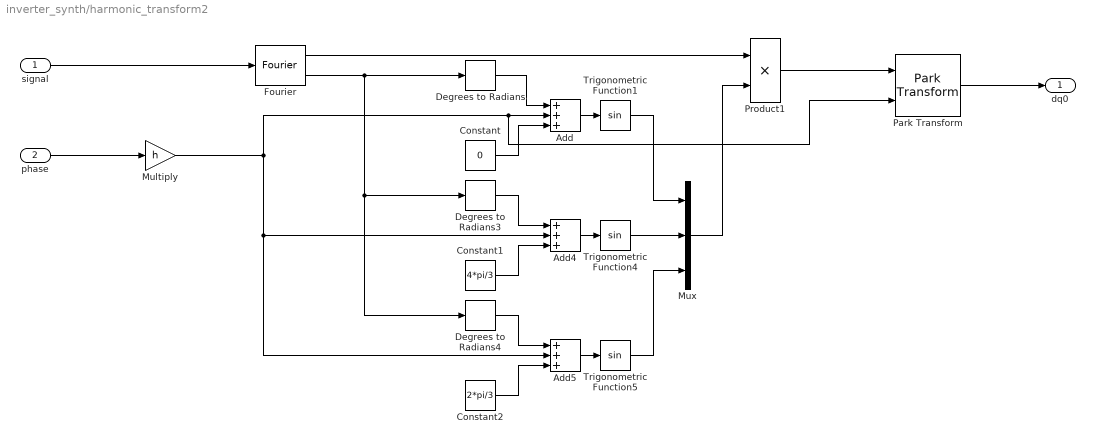
== system inverter_synth/harmonic_transform2 ==
  signal : Inport
  phase : Inport  Port=2
  Add : Sum  Inputs=+++
  Add4 : Sum  Inputs=+++
  Add5 : Sum  Inputs=+++
  Constant : Constant  Value=0
  Constant1 : Constant  Value=4*pi/3
  Constant2 : Constant  Value=2*pi/3
  Degrees to Radians : simulink_extras/Transformations/Degrees to Radians
  Degrees to Radians3 : simulink_extras/Transformations/Degrees to Radians
  Degrees to Radians4 : simulink_extras/Transformations/Degrees to Radians
  Fourier : powerlib_meascontrol/Measurements/Fourier  Freq=f0  n=h  InInit=[0, 0]  Ts=0
  Multiply : Gain  Gain=h
  Mux : Mux  Inputs=3
  Park Transform : eeTransforms/Park Transform  AxisAlignment=Q-axis  PowerInvariant=off
  Product1 : Product  RndMeth=Zero
  Trigonometric Function1 : Trigonometry
  Trigonometric Function4 : Trigonometry
  Trigonometric Function5 : Trigonometry
  dq0 : Outport
  wires:
  Add/1 -> Trigonometric Function1/1
  Multiply/1 -> Add5/2, Add4/2, Park Transform/2, Add/2
  Constant2/1 -> Add5/3
  Mux/1 -> Product1/2
  Fourier/1 -> Product1/1
  Degrees to Radians/1 -> Add/1
  Fourier/2 -> Degrees to Radians/1, Degrees to Radians3/1, Degrees to Radians4/1
  Degrees to Radians4/1 -> Add5/1
  Constant/1 -> Add/3
  Add5/1 -> Trigonometric Function5/1
  Product1/1 -> Park Transform/1
  Trigonometric Function5/1 -> Mux/3
  Trigonometric Function1/1 -> Mux/1
  Park Transform/1 -> dq0/1
  Add4/1 -> Trigonometric Function4/1
  Degrees to Radians3/1 -> Add4/1
  Constant1/1 -> Add4/3
  Trigonometric Function4/1 -> Mux/2
  signal/1 -> Fourier/1
  phase/1 -> Multiply/1
